simulink model "HANcoder_E407_TTA_CombineModel"  (R2022b)
settings: Solver=FixedStepDiscrete  StartTime=0.0  StopTime=1  FixedStep=0.001  RelTol=1e-3
PreLoadFcn:
  | librarySetup
  | eval([bdroot,'_startup']) %Calling [modelName]_startup.m
values from neighbouring files (symbols this model uses):
  ClockOn = Simulink.Parameter    [HANcoder_E407_TTA_Chris_startup.m]    (also in HANcoder_E407_TTA_CombineModel_Membership_2022a_startup.m; HANcoder_E407_TTA_CombineModel_Membership_startup.m; HANcoder_E407_TTA_CombineModel_V2_startup.m; HANcoder_E407_TTA_CombineModel_startup.m)
  controlWidth = Simulink.Parameter    [HANcoder_E407_TTA_CombineModel_Membership_2022a_startup.m]    (also in HANcoder_E407_TTA_CombineModel_Membership_startup.m; HANcoder_E407_TTA_CombineModel_V2_startup.m; HANcoder_E407_TTA_CombineModel_startup.m)
  desiredAngle = Simulink.Parameter    [HANcoder_E407_TTA_CombineModel_Membership_2022a_startup.m]    (also in HANcoder_E407_TTA_CombineModel_Membership_startup.m; HANcoder_E407_TTA_CombineModel_V2_startup.m; HANcoder_E407_TTA_CombineModel_startup.m)
  frequency_IRQ = 1000    [HANcoder_E407_TTA_Chris_startup.m]    (also in HANcoder_E407_TTA_CombineModel_Membership_2022a_startup.m; HANcoder_E407_TTA_CombineModel_Membership_startup.m; HANcoder_E407_TTA_CombineModel_V2_startup.m; HANcoder_E407_TTA_CombineModel_startup.m)
  intVal = Simulink.Parameter    [HANcoder_E407_TTA_CombineModel_Membership_2022a_startup.m]    (also in HANcoder_E407_TTA_CombineModel_Membership_startup.m; HANcoder_E407_TTA_CombineModel_V2_startup.m; HANcoder_E407_TTA_CombineModel_startup.m)
  L0b = 1    [HANcoder_E407_KinematicAngleControl_startup.m]    (also in HANcoder_E407_TTA_CombineModel_Membership_2022a_startup.m; HANcoder_E407_TTA_CombineModel_Membership_startup.m; HANcoder_E407_TTA_CombineModel_V2_startup.m; HANcoder_E407_TTA_CombineModel_startup.m)
  L0F = 3    [HANcoder_E407_KinematicAngleControl_startup.m]    (also in HANcoder_E407_TTA_CombineModel_Membership_2022a_startup.m; HANcoder_E407_TTA_CombineModel_Membership_startup.m; HANcoder_E407_TTA_CombineModel_V2_startup.m; HANcoder_E407_TTA_CombineModel_startup.m)
  L1F = 4    [HANcoder_E407_KinematicAngleControl_startup.m]    (also in HANcoder_E407_TTA_CombineModel_Membership_2022a_startup.m; HANcoder_E407_TTA_CombineModel_Membership_startup.m; HANcoder_E407_TTA_CombineModel_V2_startup.m; HANcoder_E407_TTA_CombineModel_startup.m)
  matrixRows = Simulink.Parameter    [HANcoder_E407_TTA_Chris_startup.m]    (also in HANcoder_E407_TTA_CombineModel_Membership_2022a_startup.m; HANcoder_E407_TTA_CombineModel_Membership_startup.m; HANcoder_E407_TTA_CombineModel_V2_startup.m; HANcoder_E407_TTA_CombineModel_startup.m)
  MMBS1_ID = Simulink.Parameter    [HANcoder_E407_TTA_Chris_startup.m]    (also in HANcoder_E407_TTA_CombineModel_Membership_2022a_startup.m; HANcoder_E407_TTA_CombineModel_Membership_startup.m; HANcoder_E407_TTA_CombineModel_V2_startup.m; HANcoder_E407_TTA_CombineModel_startup.m)
  propVal = Simulink.Parameter    [HANcoder_E407_TTA_CombineModel_Membership_2022a_startup.m]    (also in HANcoder_E407_TTA_CombineModel_Membership_startup.m; HANcoder_E407_TTA_CombineModel_V2_startup.m; HANcoder_E407_TTA_CombineModel_startup.m)
  ResetPosition = Simulink.Parameter    [HANcoder_E407_TTA_CombineModel_Membership_2022a_startup.m]    (also in HANcoder_E407_TTA_CombineModel_V2_startup.m)
  slotTime = Simulink.Parameter    [HANcoder_E407_TTA_Chris_startup.m]    (also in HANcoder_E407_TTA_CombineModel_Membership_2022a_startup.m; HANcoder_E407_TTA_CombineModel_Membership_startup.m; HANcoder_E407_TTA_CombineModel_V2_startup.m; HANcoder_E407_TTA_CombineModel_startup.m)
  SSTM1_ID = Simulink.Parameter    [HANcoder_E407_TTA_Chris_startup.m]    (also in HANcoder_E407_TTA_CombineModel_Membership_2022a_startup.m; HANcoder_E407_TTA_CombineModel_Membership_startup.m; HANcoder_E407_TTA_CombineModel_V2_startup.m; HANcoder_E407_TTA_CombineModel_startup.m)
  SYNC1_ID = Simulink.Parameter    [HANcoder_E407_TTA_Chris_startup.m]    (also in HANcoder_E407_TTA_CombineModel_Membership_2022a_startup.m; HANcoder_E407_TTA_CombineModel_Membership_startup.m; HANcoder_E407_TTA_CombineModel_V2_startup.m; HANcoder_E407_TTA_CombineModel_startup.m)
  TRCK1_ID1 = Simulink.Parameter    [HANcoder_E407_TTA_Chris_startup.m]    (also in HANcoder_E407_TTA_CombineModel_Membership_2022a_startup.m; HANcoder_E407_TTA_CombineModel_Membership_startup.m; HANcoder_E407_TTA_CombineModel_V2_startup.m; HANcoder_E407_TTA_CombineModel_startup.m)
  TRCK1_ID2 = Simulink.Parameter    [HANcoder_E407_TTA_Chris_startup.m]    (also in HANcoder_E407_TTA_CombineModel_Membership_2022a_startup.m; HANcoder_E407_TTA_CombineModel_Membership_startup.m; HANcoder_E407_TTA_CombineModel_V2_startup.m; HANcoder_E407_TTA_CombineModel_startup.m)
  TRCK1_ID3 = Simulink.Parameter    [HANcoder_E407_TTA_Chris_startup.m]    (also in HANcoder_E407_TTA_CombineModel_Membership_2022a_startup.m; HANcoder_E407_TTA_CombineModel_Membership_startup.m; HANcoder_E407_TTA_CombineModel_V2_startup.m; HANcoder_E407_TTA_CombineModel_startup.m)
  TRLS1_ID4 = Simulink.Parameter    [HANcoder_E407_TTA_Chris_startup.m]    (also in HANcoder_E407_TTA_CombineModel_Membership_2022a_startup.m; HANcoder_E407_TTA_CombineModel_Membership_startup.m; HANcoder_E407_TTA_CombineModel_V2_startup.m; HANcoder_E407_TTA_CombineModel_startup.m)
  TRLS1_ID5 = Simulink.Parameter    [HANcoder_E407_TTA_Chris_startup.m]    (also in HANcoder_E407_TTA_CombineModel_Membership_2022a_startup.m; HANcoder_E407_TTA_CombineModel_Membership_startup.m; HANcoder_E407_TTA_CombineModel_V2_startup.m; HANcoder_E407_TTA_CombineModel_startup.m)
  V2 = 1.3889    [HANcoder_E407_KinematicAngleControl_startup.m]    (also in HANcoder_E407_TTA_CombineModel_Membership_2022a_startup.m = 0.5; HANcoder_E407_TTA_CombineModel_Membership_startup.m = 0.5; HANcoder_E407_TTA_CombineModel_V2_startup.m = 0.5; HANcoder_E407_TTA_CombineModel_startup.m = 0.5)
undefined symbols (not defined in the file or in its folder): A2, A3, A4, CON2, CON3, CON4, D10, D4, D5
libraries: hdlsllib x95, HANcoder_STM32_Target x23, simulink_extras x4, dspstat3 x3, simulink x2, slpidlib x1
(part 5 of 5)

== system HANcoder_E407_TTA_CombineModel/HANcoder STM32 Target - E407-STM32 algorithm/Message selector/TRCK_ID3_RX/CAN receive1/Enabled Subsystem ==
  In1 : Inport
  In2 : Inport  Port=2
  In3 : Inport  Port=3
  In4 : Inport  Port=4
  In5 : Inport  Port=5
  In6 : Inport  Port=6
  In7 : Inport  Port=7
  In8 : Inport  Port=8
  Enable : EnablePort
  Out1 : Outport
  Out2 : Outport  Port=2
  Out3 : Outport  Port=3
  Out4 : Outport  Port=4
  Out5 : Outport  Port=5
  Out6 : Outport  Port=6
  Out7 : Outport  Port=7
  Out8 : Outport  Port=8
  wires:
  In8/1 -> Out8/1
  In7/1 -> Out7/1
  In6/1 -> Out6/1
  In5/1 -> Out5/1
  In4/1 -> Out4/1
  In3/1 -> Out3/1
  In2/1 -> Out2/1
  In1/1 -> Out1/1

== system HANcoder_E407_TTA_CombineModel/HANcoder STM32 Target - E407-STM32 algorithm/Message selector/TRLS_ID4_RX/CAN receive1/Enabled Subsystem ==
  In1 : Inport
  In2 : Inport  Port=2
  In3 : Inport  Port=3
  In4 : Inport  Port=4
  In5 : Inport  Port=5
  In6 : Inport  Port=6
  In7 : Inport  Port=7
  In8 : Inport  Port=8
  Enable : EnablePort
  Out1 : Outport
  Out2 : Outport  Port=2
  Out3 : Outport  Port=3
  Out4 : Outport  Port=4
  Out5 : Outport  Port=5
  Out6 : Outport  Port=6
  Out7 : Outport  Port=7
  Out8 : Outport  Port=8
  wires:
  In8/1 -> Out8/1
  In7/1 -> Out7/1
  In6/1 -> Out6/1
  In5/1 -> Out5/1
  In4/1 -> Out4/1
  In3/1 -> Out3/1
  In2/1 -> Out2/1
  In1/1 -> Out1/1

== system HANcoder_E407_TTA_CombineModel/HANcoder STM32 Target - E407-STM32 algorithm/Message selector/TRLS_ID5_RX/CAN receive1/Enabled Subsystem ==
  In1 : Inport
  In2 : Inport  Port=2
  In3 : Inport  Port=3
  In4 : Inport  Port=4
  In5 : Inport  Port=5
  In6 : Inport  Port=6
  In7 : Inport  Port=7
  In8 : Inport  Port=8
  Enable : EnablePort
  Out1 : Outport
  Out2 : Outport  Port=2
  Out3 : Outport  Port=3
  Out4 : Outport  Port=4
  Out5 : Outport  Port=5
  Out6 : Outport  Port=6
  Out7 : Outport  Port=7
  Out8 : Outport  Port=8
  wires:
  In8/1 -> Out8/1
  In7/1 -> Out7/1
  In6/1 -> Out6/1
  In5/1 -> Out5/1
  In4/1 -> Out4/1
  In3/1 -> Out3/1
  In2/1 -> Out2/1
  In1/1 -> Out1/1

== system HANcoder_E407_TTA_CombineModel/HANcoder STM32 Target - E407-STM32 algorithm/Role assignment/Subsystem2/CAN receive1/Enabled Subsystem ==
  In1 : Inport
  In2 : Inport  Port=2
  In3 : Inport  Port=3
  In4 : Inport  Port=4
  In5 : Inport  Port=5
  In6 : Inport  Port=6
  In7 : Inport  Port=7
  In8 : Inport  Port=8
  Enable : EnablePort
  Out1 : Outport
  Out2 : Outport  Port=2
  Out3 : Outport  Port=3
  Out4 : Outport  Port=4
  Out5 : Outport  Port=5
  Out6 : Outport  Port=6
  Out7 : Outport  Port=7
  Out8 : Outport  Port=8
  wires:
  In8/1 -> Out8/1
  In7/1 -> Out7/1
  In6/1 -> Out6/1
  In5/1 -> Out5/1
  In4/1 -> Out4/1
  In3/1 -> Out3/1
  In2/1 -> Out2/1
  In1/1 -> Out1/1
